simulink model "sim_integr_old"  (R2021b)
settings: Solver=ode8  StartTime=0.0  StopTime=2  FixedStep=1e-6  RelTol=1e-3
settings Model: Creator=isaac  LastModifiedBy=isaac

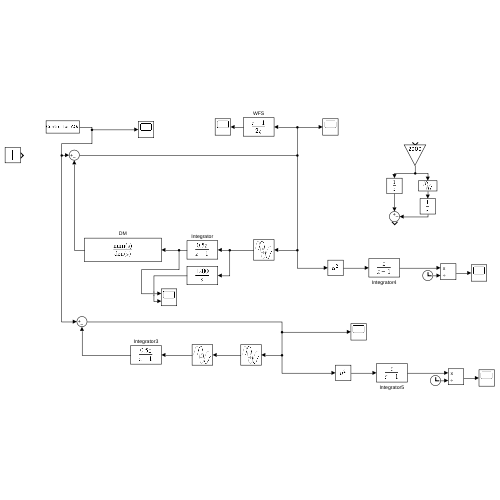
[thumbnail: Simulink's stored preview of the top-level diagram]
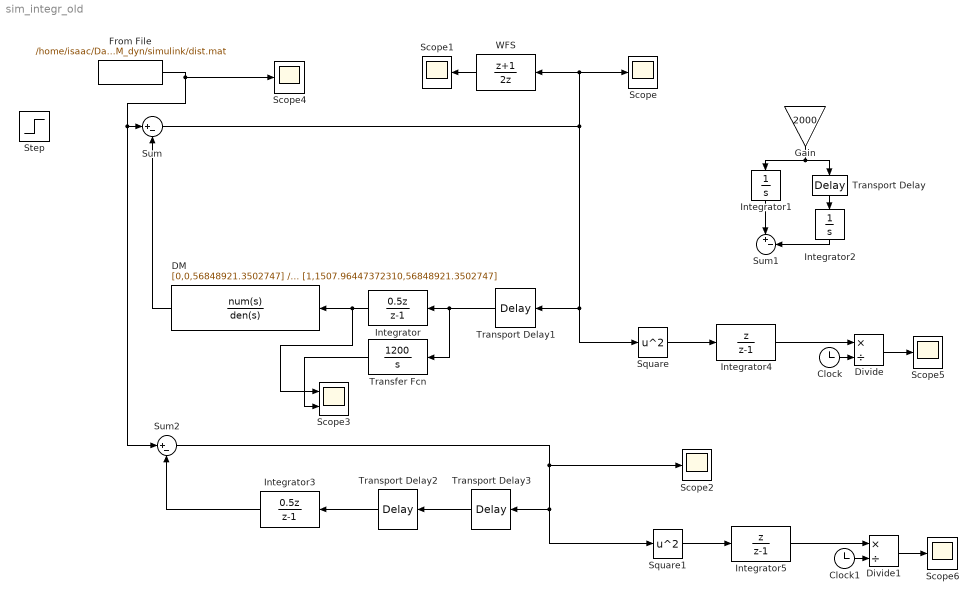
== system sim_integr_old ==
  Clock : Clock
  Clock1 : Clock
  DM : TransferFcn  Tag=DM  Numerator=[0,0,56848921.3502747]  Denominator=[1,1507.96447372310,56848921.3502747]
  Divide : Product  Inputs=*/
  Divide1 : Product  Inputs=*/
  From File : FromFile  FileName=/home/isaac/Data-Driven-Control-for-AO/DM_dyn/simulink/dist.mat
  Gain : Gain  Gain=2000
  Integrator : DiscreteTransferFcn  Numerator=[0.5 0]  Denominator=[1 -1]  SampleTime=0.0005
  Integrator1 : Integrator
  Integrator2 : Integrator
  Integrator3 : DiscreteTransferFcn  Numerator=[0.5 0]  Denominator=[1 -1]  SampleTime=0.0005
  Integrator4 : DiscreteTransferFcn  Numerator=[1 0]  Denominator=[1 -1]
  Integrator5 : DiscreteTransferFcn  Numerator=[1 0]  Denominator=[1 -1]
  Scope{,1..2,4..6} (6 alike) : Scope
  Scope3 : Scope  NumInputPorts=2
  Square : Math  Operator=square  SaturateOnIntegerOverflow=on
  Square1 : Math  Operator=square  SaturateOnIntegerOverflow=on
  Step : Step  Before=1  SampleTime=0
  Sum : Sum  Inputs=|+-
  Sum1 : Sum  Inputs=|+-
  Sum2 : Sum  Inputs=|+-
  Transfer Fcn : TransferFcn  Numerator=[1200]  Denominator=[1 0]
  Transport Delay : TransportDelay  DelayTime=0.0005
  Transport Delay1 : TransportDelay  DelayTime=0.00065
  Transport Delay2 : TransportDelay  DelayTime=0.00065
  Transport Delay3 : TransportDelay  DelayTime=0.0000001
  WFS : DiscreteTransferFcn  Numerator=[1 1]  Denominator=[2 0]
  wires:
  WFS/1 -> Scope1/1
  DM/1 -> Sum/2
  Transport Delay1/1 -> Transfer Fcn/1, Integrator/1
  Integrator/1 -> DM/1, Scope3/1
  Transfer Fcn/1 -> Scope3/2
  From File/1 -> Sum2/1, Sum/1, Scope4/1
  Transport Delay/1 -> Integrator2/1
  Integrator2/1 -> Sum1/2
  Integrator1/1 -> Sum1/1
  Gain/1 -> Integrator1/1, Transport Delay/1
  Sum/1 -> Square/1, Transport Delay1/1, Scope/1, WFS/1
  Transport Delay2/1 -> Integrator3/1
  Integrator3/1 -> Sum2/2
  Clock/1 -> Divide/2
  Divide/1 -> Scope5/1
  Integrator4/1 -> Divide/1
  Square/1 -> Integrator4/1
  Integrator5/1 -> Divide1/1
  Sum2/1 -> Scope2/1, Transport Delay3/1, Square1/1
  Divide1/1 -> Scope6/1
  Square1/1 -> Integrator5/1
  Clock1/1 -> Divide1/2
  Transport Delay3/1 -> Transport Delay2/1
